simulink subsystem "DiscreteController2ndDegree"  (R2024b)
settings: Solver=VariableStepAuto  StartTime=0.0  StopTime=10.0  RelTol=1e-3
undefined symbols (not defined in the file or in its folder): P, Q
settings Model: Creator=lukiq  LastModifiedBy=lukiq

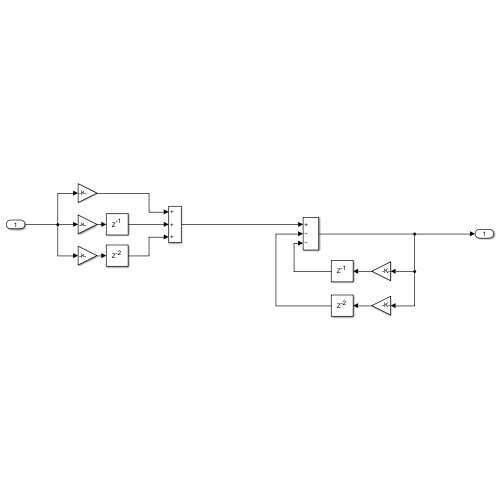
[thumbnail: Simulink's stored preview of the top-level diagram]
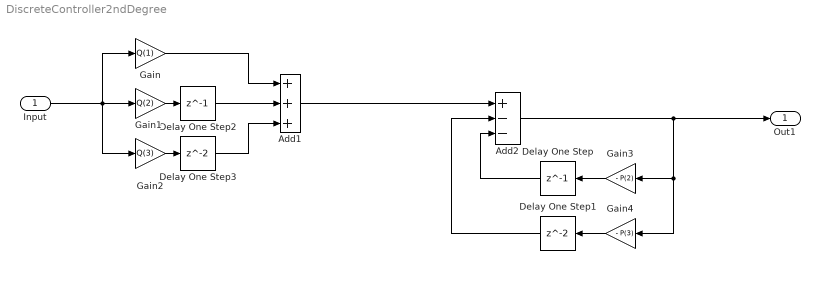
== system DiscreteController2ndDegree ==
  Input : Inport
  Add1 : Sum  Inputs=+++
  Add2 : Sum  Inputs=+--
  Delay One Step : Delay  DelayLength=1
  Delay One Step1 : Delay
  Delay One Step2 : Delay  DelayLength=1
  Delay One Step3 : Delay
  Gain : Gain  Gain=Q(1)
  Gain1 : Gain  Gain=Q(2)
  Gain2 : Gain  Gain=Q(3)
  Gain3 : Gain  Gain=- P(2)
  Gain4 : Gain  Gain=- P(3)
  Out1 : Outport
  wires:
  Add2/1 -> Out1/1, Gain3/1, Gain4/1
  Delay One Step/1 -> Add2/3
  Gain4/1 -> Delay One Step1/1
  Add1/1 -> Add2/1
  Input/1 -> Gain2/1, Gain1/1, Gain/1
  Gain2/1 -> Delay One Step3/1
  Gain1/1 -> Delay One Step2/1
  Delay One Step1/1 -> Add2/2
  Gain3/1 -> Delay One Step/1
  Gain/1 -> Add1/1
  Delay One Step3/1 -> Add1/3
  Delay One Step2/1 -> Add1/2
